simulink model "calculate_wave"  (R2023a)
settings: Solver=VariableStepAuto  StartTime=0.0  StopTime=10.0  MaxStep=0.01  RelTol=1e-3
undefined symbols (not defined in the file): freq
settings Model: Creator=fy153  LastModifiedBy=fy153

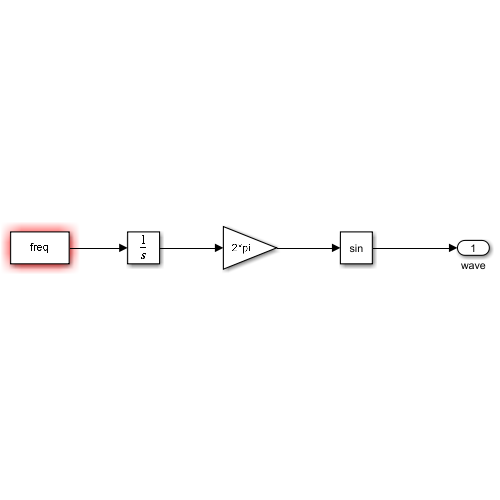
[thumbnail: Simulink's stored preview of the top-level diagram]
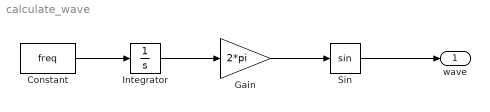
== system calculate_wave ==
  Constant : Constant  Value=freq
  Gain : Gain  Gain=2*pi
  Integrator : Integrator
  Sin : Trigonometry
  wave : Outport
  wires:
  Constant/1 -> Integrator/1
  Gain/1 -> Sin/1
  Integrator/1 -> Gain/1
  Sin/1 -> wave/1
